simulink subsystem "harmonicFeatures"  (R2021a)
settings: Solver=VariableStepAuto  StartTime=0.0  StopTime=10.0  RelTol=1e-3
libraries: dspstat3 x1
settings Model: Creator=trevor  LastModifiedBy=trevvvy
settings SolverCC: AlgebraicLoopSolver=TrustRegion
settings DebuggingCC: SFMachineParentedDataDiag=warning

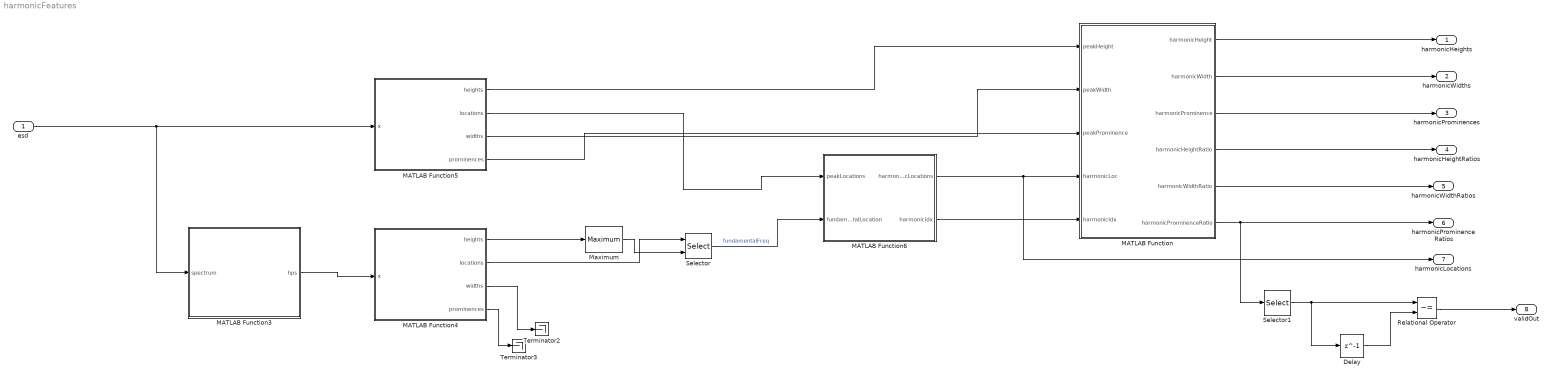
== system harmonicFeatures ==
  esd : Inport
  Delay : Delay  DelayLength=1
  MATLAB Function : MATLAB Function  TreatAsAtomicUnit=on
  MATLAB Function3 : MATLAB Function  TreatAsAtomicUnit=on
  MATLAB Function4 : MATLAB Function  TreatAsAtomicUnit=on
  MATLAB Function5 : MATLAB Function  TreatAsAtomicUnit=on
  MATLAB Function6 : MATLAB Function  TreatAsAtomicUnit=on
  Maximum : dspstat3/Maximum  operation=maximum  fcn=Index  indexBase=One  operateOver=Each row  Dimension=1  InputProcessing=Columns as channels (frame based)  reset=None  roiEnable=off  roiType=Rectangles  roiPortion=Entire ROI  roiOutput=Individual statistics for each ROI  roiFlag=off  roundingMode=Floor  overflowMode=off  accumDataTypeStr=Inherit: Same as product output  accumLastDataTypeStr=Inherit: Same as product output
  Relational Operator : RelationalOperator  Operator=~=  OutDataTypeStr=boolean  RndMeth=Simplest
  Selector : Selector  InputPortWidth=85  IndexOptions=Index vector (port)  Indices=[1 3]  OutputSizes=1
  Selector1 : Selector  InputPortWidth=3  IndexOptions=Index vector (dialog)  Indices=1  OutputSizes=1
  Terminator2 : Terminator
  Terminator3 : Terminator
  harmonicHeights : Outport
  harmonicWidths : Outport  Port=2
  harmonicProminences : Outport  Port=3
  harmonicHeightRatios : Outport  Port=4
  harmonicWidthRatios : Outport  Port=5
  harmonicProminenceRatios : Outport  Port=6
  harmonicLocations : Outport  Port=7
  validOut : Outport  Port=8
  wires:
  esd/1 -> MATLAB Function3/1(spectrum), MATLAB Function5/1(x)
  MATLAB Function4/2(locations) -> Selector/1
  MATLAB Function4/3(widths) -> Terminator2/1
  MATLAB Function4/4(prominences) -> Terminator3/1
  MATLAB Function3/1(hps) -> MATLAB Function4/1(x)
  MATLAB Function4/1(heights) -> Maximum/1
  Maximum/1 -> Selector/2
  Selector/1 -> MATLAB Function6/2(fundamentalLocation)  "fundamentalFreq"
  MATLAB Function6/1(harmonicLocations) -> MATLAB Function/4(harmonicLoc), harmonicLocations/1
  MATLAB Function6/2(harmonicIdx) -> MATLAB Function/5(harmonicIdx)
  MATLAB Function5/2(locations) -> MATLAB Function6/1(peakLocations)
  MATLAB Function5/3(widths) -> MATLAB Function/2(peakWidth)
  MATLAB Function5/4(prominences) -> MATLAB Function/3(peakProminence)
  MATLAB Function5/1(heights) -> MATLAB Function/1(peakHeight)
  MATLAB Function/1(harmonicHeight) -> harmonicHeights/1
  MATLAB Function/2(harmonicWidth) -> harmonicWidths/1
  MATLAB Function/3(harmonicProminence) -> harmonicProminences/1
  MATLAB Function/4(harmonicHeightRatio) -> harmonicHeightRatios/1
  MATLAB Function/5(harmonicWidthRatio) -> harmonicWidthRatios/1
  MATLAB Function/6(harmonicProminenceRatio) -> harmonicProminenceRatios/1, Selector1/1
  Relational Operator/1 -> validOut/1
  Delay/1 -> Relational Operator/2
  Selector1/1 -> Relational Operator/1, Delay/1

== matlab function harmonicFeatures/MATLAB Function ==
  settings: fimath=fimath('RoundingMethod', 'Floor','OverflowAction', 'Wrap','ProductMode', 'FullPrecision', 'SumMode', 'FullPrecision')
  data: peakHeight input; harmonicHeight output; peakWidth input; peakProminence input; harmonicLoc input; harmonicIdx input; harmonicWidth output; harmonicProminence output; harmonicHeightRatio output; harmonicWidthRatio output; harmonicProminenceRatio output
function [harmonicHeight, harmonicWidth, harmonicProminence, harmonicHeightRatio, harmonicWidthRatio, harmonicProminenceRatio] = extractHarmonicFeatures(peakHeight, peakWidth, peakProminence, harmonicLoc, harmonicIdx)
% extractHarmonicFeatures extract features related to harmonics in the PSD.
%
%   features = extractHarmonicFeatures(psd, nHarmonics) extracts features from
%   the power spectral density, psd, for nHarmonics harmonics. psd is a
%   one-sided power spectral density magnitude, i.e. abs(fft(X)).^2. 
%
%   The extracted features for each harmonic are:
%       'HarmonicHeight'            - The height of the harmonic
%       'HarmonicLoc'               - The harmonic location (frequency bin)
%       'HarmonicWidth'             - The harmonic's half-prominence peak width
%       'HarmonicProminence'        - The harmonic's prominence
%
%   The extracted features for all combinations of n-choose-2 harmonics are:
%       'HarmonicHeightRatio'       - The ratio between harmonic heights
%       'HarmonicWidthRatio'        - The ratio between harmonic widths
%       'HarmonicProminenceRatio'   - The ratio between harmonic prominences

% SPDX-License-Identifier: BSD-3-Clause

% TODO: make nBins an input parameter

%#codegen



harmonicCombinations = [1 2; 1 3; 2 3];
% harmonicCombinations = nchoosek(1:nHarmonics, 2);

harmonicHeight = zeros(1, 3, 'like', peakHeight);
harmonicWidth = zeros(1, 3, 'like', peakWidth);
harmonicProminence = zeros(1, 3, 'like', peakProminence);
harmonicHeightRatio = zeros(1, 3, 'like', peakHeight);
harmonicWidthRatio = zeros(1, 3, 'like', peakWidth);
harmonicProminenceRatio = zeros(1, 3, 'like', peakProminence);



% Get features for the harmonics. If a harmonic wasn't found, harmonicIdx
% will be 0. All related features to be 0 if the harmonic wasn't found.
for j = 1:numel(harmonicIdx)
    if harmonicIdx(j) ~= 0
        harmonicWidth(j) = peakWidth(harmonicIdx(j));
        harmonicProminence(j) = peakProminence(harmonicIdx(j));
        harmonicHeight(j) = peakHeight(harmonicIdx(j));
    end
end

% Compute feature ratios for all n-choose-2 combinations of harmonics
for n = 1:3
    % Get the harmonic numbers we are taking a ratio of
    harmonic1 = harmonicCombinations(n, 1);
    harmonic2 = harmonicCombinations(n, 2);

    if harmonicHeight(harmonic2) ~= 0
        harmonicHeightRatio(n) = harmonicHeight(harmonic1) / harmonicHeight(harmonic2);
    else
        harmonicHeightRatio(n) = 0;
    end

    if harmonicWidth(harmonic2) ~= 0
        harmonicWidthRatio(n) = harmonicWidth(harmonic1) / harmonicWidth(harmonic2);
    else
        harmonicWidthRatio(n) = 0;
    end

    if harmonicProminence(harmonic2) ~= 0
        harmonicProminenceRatio(n) = harmonicProminence(harmonic1) / harmonicProminence(harmonic2);
    else
        harmonicProminenceRatio(n) = 0;
    end
end



end

== matlab function harmonicFeatures/MATLAB Function4 ==
  settings: fimath=fimath('RoundingMethod', 'Floor','OverflowAction', 'Wrap','ProductMode', 'FullPrecision', 'SumMode', 'FullPrecision')
  data: x input; heights output; locations output; widths output; prominences output
function [heights, locations, widths, prominences] = findPeaks(x)
% findPeaks Find local maxima in a 1D signal
%
%   A peak is defined as any sample that is larger than it's neighbors.
%
%   [heights, locations, widths, prominences] = findPeaks(x) finds all peaks in
%   the signal x. It returns the height, location, width, and prominence of each
%   peak. The peak widths are measured at half-prominence height.
%
%   For plateaus, findPeaks returns the first index of the plateau.

% Much of the code contained here was ported from scipy's find_peaks
% implementation. scipy is licensed under the BSD 3-clause license.
% Copyright (c) 2001-2002 Enthought, Inc. 2003-2022, SciPy Developers
% Copyright (c) 2022 Trevor Vannoy
% SPDX-License-Identifier: BSD-3-Clause

%#codegen

locations = localMaxima1d(x);

heights = zeros(size(locations), 'like', x);
for i = 1:numel(locations)
    if locations(i) ~= 0
        heights(i) = x(locations(i));
    end
end

[prominences, leftBases, rightBases] = peakProminence(x, locations);

widths = peakWidths(x, locations, prominences, leftBases, rightBases);


end

function [locations] = localMaxima1d(x)
% localMaxima1d Find local maxima in a 1D array
%
% Inputs:
%   - x: the signal in which to find maxima
%
% Outputs:
%   - locations: the indices of each maxima/peak

% preallocate; there can't be more maxima than half the size of x
locations = zeros(1, floor(numel(x)/2), 'int32');
nPeaksIdx = 1;


% the first sample can't be a maxima, so we start at 2
iMin = 2;
% last sample can't be a maxima either
iMax = numel(x) - 1;

for i =  iMin:iMax
    % if the previous sample is smaller and the next sample is at least
    % as small, we've found a peak. 
    if x(i - 1) < x(i)

        % if the next sample is equal to the current one, we've hit a plateau;
        % we return the beginning of the plateau as the peak location, which
        % is consistent with MATLAB's findpeaks behavior.
        if x(i + 1) <= x(i)
            locations(nPeaksIdx) = i;
            nPeaksIdx(:) = nPeaksIdx + 1;
        end
    end

end
end

function [prominences, leftBases, rightBases] = peakProminence(x, locations)
% peakProminence Calculate the prominence of each peak in a signal.
%
% Inputs:
%   - x: the signal
%   - locations: the locations of each peak in x
%
% Outputs:
%   - prominences: the prominence for each peak
%   - leftBases: the left base of each peak
%   - rightBases: the right base of each peak

% preallocate
prominences = zeros(size(locations), 'like', x);
leftBases = zeros(size(locations), 'like', locations);
rightBases = zeros(size(locations), 'like', locations);

iMin = cast(1, 'like', locations);
iMax = cast(numel(x), 'like', locations);

for peakNum = 1:numel(locations)
    % locations == 0 means there wasn't a peak, so skip those
    if locations(peakNum) ~= 0
        location = locations(peakNum);

        % Find the left base in interval [iMin, location]
        leftBases(peakNum) = location;
        i = location;
        leftMin = x(location);

        leftBorder = iMin;
        for i = iMin:iMax
            if i < location
                if x(i) >= x(location)
                    leftBorder = i;
                end
            end
        end
        for i = iMax:-1:iMin
            if i <= location && i >= leftBorder
                if x(i) < leftMin
                    leftMin = x(i);
                    leftBases(peakNum) = i;
                end
            end
        end

        % Find the right base in interval [location, iMax]
        rightBases(peakNum) = location;
        i = location;
        rightMin = x(location);

        rightBorder = iMax;
        for i = iMax:-1:iMin
            if i > location
                if x(i) >= x(location)
                    rightBorder = i;
                end
            end
        end
        for i = iMax:-1:iMin
            if i <= rightBorder && i >= location
                if x(i) < rightMin
                    rightMin = x(i);
                    rightBases(peakNum) = i;
                end
            end
        end

        prominences(peakNum) = x(location) - max(leftMin, rightMin);
    end
end
end

function widths = peakWidths(x, locations, prominences, leftBases, rightBases)
% peakWidths Calculate the half-prominence width of each peak
%
% Inputs:
%   - x: the signal
%   - locations: the locations of each peak in x
%   - prominences: the prominence for each peak
%   - leftBases: the left base of each peak
%   - rightBases: the right base of each peak
%
% Outputs:
%   - widths: the width for each peak

% widths are measured at half-prominence height
relHeight = 0.5;

widths = zeros(size(locations), 'like', x);

iMin = cast(1, 'like', locations);
iMax = cast(numel(x), 'like', locations);

for peakNum = 1:numel(locations)
    % locations == 0 means there wasn't a peak, so skip those
    if locations(peakNum) ~= 0
        leftBase = leftBases(peakNum);
        rightBase = rightBases(peakNum);
        location = locations(peakNum);

        height = x(location) - prominences(peakNum) * relHeight;

        % Find intersection point on left side
        leftIp = cast(iMin, 'like', x);
        done = false;
        for i = iMax:-1:iMin
            if i <= location && i >= leftBase
                if ~done
                    if x(i) <= height
                        done = true;
                        leftIp = cast(i, 'like', x);
                    end
                end
            end
        end
        
        if x(leftIp) < height
            % Interpolate if true intersection height is between samples
            leftIp(:) = leftIp + (height - x(leftIp)) / (x(leftIp + 1) - x(leftIp));
        end

        % Find intersection point on right side
        rightIp = cast(iMax, 'like', x);
        done = false;
        for i = iMin:iMax
            if i >= location && i <= rightBase
                if ~done
                    if x(i) <= height
                        done = true;
                        rightIp = cast(i, 'like', x);
                    end
                end
            end
        end

        if x(rightIp) < height
            % Interpolate if true intersection height is between samples
            rightIp(:) = rightIp - (height - x(rightIp)) / (x(rightIp - 1) - x(rightIp));
        end

        widths(peakNum) = rightIp - leftIp;
    end
end
end

== matlab function harmonicFeatures/MATLAB Function3 ==
  settings: fimath=fimath('RoundingMethod', 'Floor','OverflowAction', 'Wrap','ProductMode', 'FullPrecision', 'SumMode', 'FullPrecision')
  data: spectrum input; hps output
function hps = harmonicProductSpectrum(spectrum)
% harmonicProductSpectrum compute the harmonic product spectrum of a one-sided
% spectrum or PSD
%
%   hps = harmonicProductSpectrum(spectrum, nSpectra) computes the haromnic
%   product spectrum. spectrum is a one-sided magnitude spectrum or one-sided
%   power spectral density. nSpectra determines the the number of spectral
%   copies to use when computing the harmonic product spectrum.

% SPDX-License-Identifier: BSD-3-Clause

%#codegen

cols = floor(512/3);


hps = spectrum(:,1:cols);
hps(:) = hps .* spectrum(:,1:2:2*cols);
hps(:) = hps .* spectrum(:,1:3:3*cols);

end

== matlab function harmonicFeatures/MATLAB Function5 ==
  settings: fimath=fimath('RoundingMethod', 'Floor','OverflowAction', 'Wrap','ProductMode', 'FullPrecision', 'SumMode', 'FullPrecision')
  data: x input; heights output; locations output; widths output; prominences output
function [heights, locations, widths, prominences] = findPeaks(x)
% findPeaks Find local maxima in a 1D signal
%
%   A peak is defined as any sample that is larger than it's neighbors.
%
%   [heights, locations, widths, prominences] = findPeaks(x) finds all peaks in
%   the signal x. It returns the height, location, width, and prominence of each
%   peak. The peak widths are measured at half-prominence height.
%
%   For plateaus, findPeaks returns the first index of the plateau.

% Much of the code contained here was ported from scipy's find_peaks
% implementation. scipy is licensed under the BSD 3-clause license.
% Copyright (c) 2001-2002 Enthought, Inc. 2003-2022, SciPy Developers
% Copyright (c) 2022 Trevor Vannoy
% SPDX-License-Identifier: BSD-3-Clause

%#codegen

locations = localMaxima1d(x);

heights = zeros(size(locations), 'like', x);
for i = 1:numel(locations)
    if locations(i) ~= 0
        heights(i) = x(locations(i));
    end
end

[prominences, leftBases, rightBases] = peakProminence(x, locations);

widths = peakWidths(x, locations, prominences, leftBases, rightBases);


end

function [locations] = localMaxima1d(x)
% localMaxima1d Find local maxima in a 1D array
%
% Inputs:
%   - x: the signal in which to find maxima
%
% Outputs:
%   - locations: the indices of each maxima/peak

% preallocate; there can't be more maxima than half the size of x
locations = zeros(1, floor(numel(x)/2), 'int32');
nPeaksIdx = 1;


% the first sample can't be a maxima, so we start at 2
iMin = 2;
% last sample can't be a maxima either
iMax = numel(x) - 1;

for i =  iMin:iMax
    % if the previous sample is smaller and the next sample is at least
    % as small, we've found a peak. 
    if x(i - 1) < x(i)

        % if the next sample is equal to the current one, we've hit a plateau;
        % we return the beginning of the plateau as the peak location, which
        % is consistent with MATLAB's findpeaks behavior.
        if x(i + 1) <= x(i)
            locations(nPeaksIdx) = i;
            nPeaksIdx(:) = nPeaksIdx + 1;
        end
    end

end
end

function [prominences, leftBases, rightBases] = peakProminence(x, locations)
% peakProminence Calculate the prominence of each peak in a signal.
%
% Inputs:
%   - x: the signal
%   - locations: the locations of each peak in x
%
% Outputs:
%   - prominences: the prominence for each peak
%   - leftBases: the left base of each peak
%   - rightBases: the right base of each peak

% preallocate
prominences = zeros(size(locations), 'like', x);
leftBases = zeros(size(locations), 'like', locations);
rightBases = zeros(size(locations), 'like', locations);

iMin = cast(1, 'like', locations);
iMax = cast(numel(x), 'like', locations);

for peakNum = 1:numel(locations)
    % locations == 0 means there wasn't a peak, so skip those
    if locations(peakNum) ~= 0
        location = locations(peakNum);

        % Find the left base in interval [iMin, location]
        leftBases(peakNum) = location;
        i = location;
        leftMin = x(location);

        leftBorder = iMin;
        for i = iMin:iMax
            if i < location
                if x(i) >= x(location)
                    leftBorder = i;
                end
            end
        end
        for i = iMax:-1:iMin
            if i <= location && i >= leftBorder
                if x(i) < leftMin
                    leftMin = x(i);
                    leftBases(peakNum) = i;
                end
            end
        end

        % Find the right base in interval [location, iMax]
        rightBases(peakNum) = location;
        i = location;
        rightMin = x(location);

        rightBorder = iMax;
        for i = iMax:-1:iMin
            if i > location
                if x(i) >= x(location)
                    rightBorder = i;
                end
            end
        end
        for i = iMax:-1:iMin
            if i <= rightBorder && i >= location
                if x(i) < rightMin
                    rightMin = x(i);
                    rightBases(peakNum) = i;
                end
            end
        end

        prominences(peakNum) = x(location) - max(leftMin, rightMin);
    end
end
end

function widths = peakWidths(x, locations, prominences, leftBases, rightBases)
% peakWidths Calculate the half-prominence width of each peak
%
% Inputs:
%   - x: the signal
%   - locations: the locations of each peak in x
%   - prominences: the prominence for each peak
%   - leftBases: the left base of each peak
%   - rightBases: the right base of each peak
%
% Outputs:
%   - widths: the width for each peak

% widths are measured at half-prominence height
relHeight = 0.5;

widths = zeros(size(locations), 'like', x);

iMin = cast(1, 'like', locations);
iMax = cast(numel(x), 'like', locations);

for peakNum = 1:numel(locations)
    % locations == 0 means there wasn't a peak, so skip those
    if locations(peakNum) ~= 0
        leftBase = leftBases(peakNum);
        rightBase = rightBases(peakNum);
        location = locations(peakNum);

        height = x(location) - prominences(peakNum) * relHeight;

        % Find intersection point on left side
        leftIp = cast(iMin, 'like', x);
        done = false;
        for i = iMax:-1:iMin
            if i <= location && i >= leftBase
                if ~done
                    if x(i) <= height
                        done = true;
                        leftIp = cast(i, 'like', x);
                    end
                end
            end
        end
        
        if x(leftIp) < height
            % Interpolate if true intersection height is between samples
            leftIp(:) = leftIp + (height - x(leftIp)) / (x(leftIp + 1) - x(leftIp));
        end

        % Find intersection point on right side
        rightIp = cast(iMax, 'like', x);
        done = false;
        for i = iMin:iMax
            if i >= location && i <= rightBase
                if ~done
                    if x(i) <= height
                        done = true;
                        rightIp = cast(i, 'like', x);
                    end
                end
            end
        end

        if x(rightIp) < height
            % Interpolate if true intersection height is between samples
            rightIp(:) = rightIp - (height - x(rightIp)) / (x(rightIp - 1) - x(rightIp));
        end

        widths(peakNum) = rightIp - leftIp;
    end
end
end

== matlab function harmonicFeatures/MATLAB Function6 ==
  settings: fimath=fimath('RoundingMethod', 'Floor','OverflowAction', 'Wrap','ProductMode', 'FullPrecision', 'SumMode', 'FullPrecision')
  data: peakLocations input; harmonicLocations output; harmonicIdx output; fundamentalLocation input
function [harmonicLocations, harmonicIdx] = findHarmonics(peakLocations, fundamentalLocation)

nHarmonics = 3;
nBins = 2;

harmonicLocations = zeros(nHarmonics, 1, 'like', peakLocations);
harmonicFreqs = zeros(nHarmonics, 1, 'like', peakLocations);
harmonicIdx = zeros(nHarmonics, 1, 'like', peakLocations);

% MATLAB indexing starts at one, so we need to remove 1 from the frequency
% location to get the actual frequency index/bin
fundamentalFreq = fundamentalLocation - 1;
peakFreqs = peakLocations - 1;

for i = 1:numel(peakLocations)
    for harmonicNum = 1:nHarmonics
        harmonic = fundamentalFreq * harmonicNum;

        freqDiff = abs(peakFreqs(i) - harmonic);
        if freqDiff <= nBins
            % the peak is within range of the theoretical harmonic frequency.
            if harmonicFreqs(harmonicNum) ~= 0
                % if a potential harmonic has already been found, check if the
                % new candidate is closer than the previous candidate. Keep the 
                % candidate that is closest to the theoretical harmonic.
                previousFreqDiff = abs(harmonicFreqs(harmonicNum) - harmonic);
                if freqDiff < previousFreqDiff
                    harmonicFreqs(harmonicNum) = peakFreqs(i);
                    harmonicIdx(harmonicNum) = i;
                end
            else
                % this is the first harmonic candidate we've found
                harmonicFreqs(harmonicNum) = peakFreqs(i);
                harmonicIdx(harmonicNum) = i;
            end
        end
    end
end

harmonicLocations = harmonicFreqs + 1;

% When we don't find a particular harmonic, e.g. harmonic 2 because the
% the harmonics are all odd, we want to return a 0 (or a NaN) to indicate that 
% no harmonic was found at that location.
for i = 1:nHarmonics
    if harmonicLocations(i) == 1
        harmonicLocations(i) = 0;
    end
end
